simulink library "Equations_of_Motion"  (R2024a)
settings: Solver=VariableStepAuto  StartTime=0.0  StopTime=10.0  RelTol=1e-3
undefined symbols (not defined in the file): g
settings Model: Creator=mahariansyah  LastModifiedBy=mahariansyah

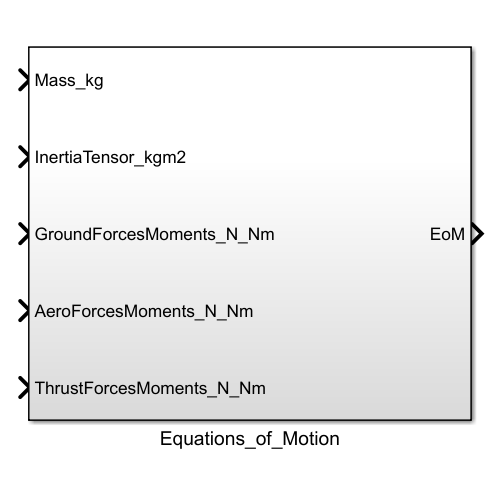
[thumbnail: Simulink's stored preview of the top-level diagram]
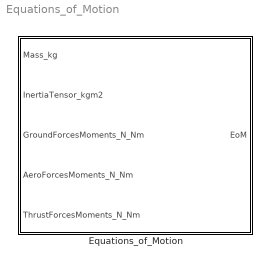
== system Equations_of_Motion ==
  Equations_of_Motion : Subsystem

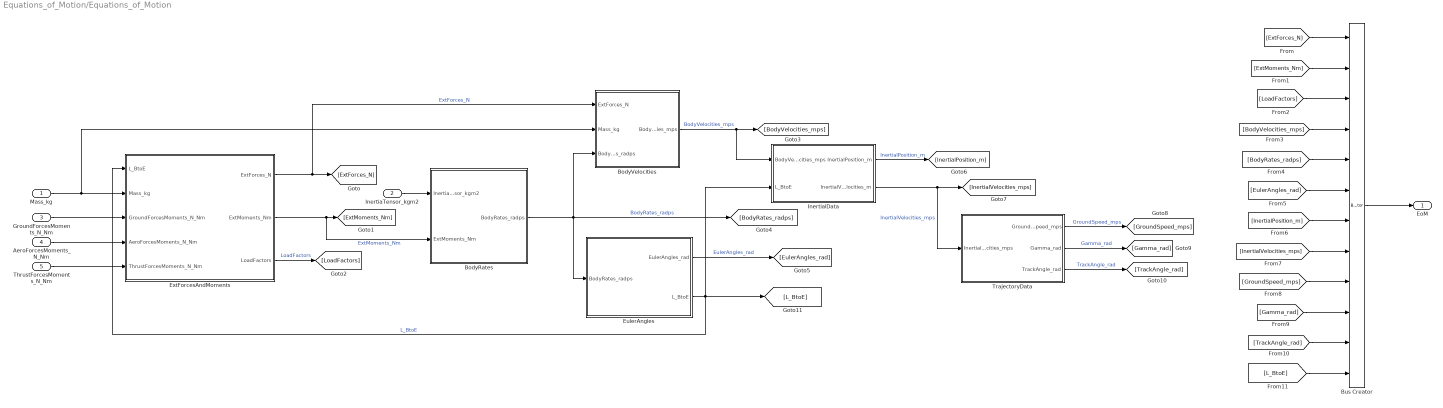
== system Equations_of_Motion/Equations_of_Motion ==
  Mass_kg : Inport
  InertiaTensor_kgm2 : Inport  Port=2
  GroundForcesMoments_N_Nm : Inport  Port=3
  AeroForcesMoments_N_Nm : Inport  Port=4
  ThrustForcesMoments_N_Nm : Inport  Port=5
  BodyRates : Subsystem
  BodyVelocities : Subsystem
  Bus Creator : BusCreator  Inputs=12
  EulerAngles : Subsystem
  ExtForcesAndMoments : Subsystem
  InertialData : Subsystem
  TrajectoryData : Subsystem
  EoM : Outport
  wires:
  [L_BtoE] -> Bus Creator/12
  ExtForcesAndMoments/1(ExtForces_N) -> [ExtForces_N], BodyVelocities/1(ExtForces_N)  "ExtForces_N"
  InertiaTensor_kgm2/1 -> BodyRates/1(InertiaTensor_kgm2)
  Mass_kg/1 -> BodyVelocities/2(Mass_kg), ExtForcesAndMoments/2(Mass_kg)
  Bus Creator/1 -> EoM/1
  BodyVelocities/1(BodyVelocities_mps) -> [BodyVelocities_mps], InertialData/1(BodyVelocities_mps)  "BodyVelocities_mps"
  EulerAngles/2(L_BtoE) -> InertialData/2(L_BtoE), ExtForcesAndMoments/1(L_BtoE), [L_BtoE]  "L_BtoE"
  BodyRates/1(BodyRates_radps) -> BodyVelocities/3(BodyRates_radps), EulerAngles/1(BodyRates_radps), [BodyRates_radps]  "BodyRates_radps"
  [GroundSpeed_mps] -> Bus Creator/9
  AeroForcesMoments_N_Nm/1 -> ExtForcesAndMoments/4(AeroForcesMoments_N_Nm)
  ExtForcesAndMoments/2(ExtMoments_Nm) -> [ExtMoments_Nm], BodyRates/2(ExtMoments_Nm)  "ExtMoments_Nm"
  [TrackAngle_rad] -> Bus Creator/11
  GroundForcesMoments_N_Nm/1 -> ExtForcesAndMoments/3(GroundForcesMoments_N_Nm)
  [BodyRates_radps] -> Bus Creator/5
  [ExtForces_N] -> Bus Creator/1
  [ExtMoments_Nm] -> Bus Creator/2
  [BodyVelocities_mps] -> Bus Creator/4
  [InertialPosition_m] -> Bus Creator/7
  [InertialVelocities_mps] -> Bus Creator/8
  TrajectoryData/2(Gamma_rad) -> [Gamma_rad]  "Gamma_rad"
  ThrustForcesMoments_N_Nm/1 -> ExtForcesAndMoments/5(ThrustForcesMoments_N_Nm)
  InertialData/2(InertialVelocities_m) -> [InertialVelocities_mps], TrajectoryData/1(InertialVelocities_mps)  "InertialVelocities_mps"
  EulerAngles/1(EulerAngles_rad) -> [EulerAngles_rad]  "EulerAngles_rad"
  [LoadFactors] -> Bus Creator/3
  [EulerAngles_rad] -> Bus Creator/6
  [Gamma_rad] -> Bus Creator/10
  TrajectoryData/3(TrackAngle_rad) -> [TrackAngle_rad]  "TrackAngle_rad"
  TrajectoryData/1(GroundSpeed_mps) -> [GroundSpeed_mps]  "GroundSpeed_mps"
  ExtForcesAndMoments/3(LoadFactors) -> [LoadFactors]  "LoadFactors"
  InertialData/1(InertialPosition_m) -> [InertialPosition_m]  "InertialPosition_m"

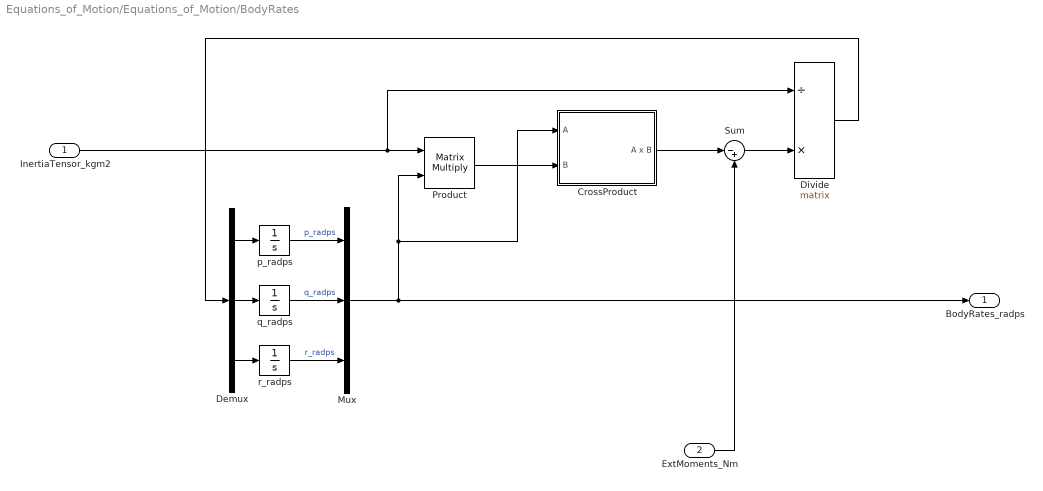
== system Equations_of_Motion/Equations_of_Motion/BodyRates ==
  InertiaTensor_kgm2 : Inport
  ExtMoments_Nm : Inport  Port=2
  CrossProduct : Subsystem
  Demux : Demux  Outputs=3
  Divide : Product  Inputs=/*  Multiplication=Matrix(*)
  Mux : Mux  Inputs=3
  Product : Product  Multiplication=Matrix(*)
  Sum : Sum  Inputs=|-+
  p_radps : Integrator  ContinuousStateAttributes='p_radps'
  q_radps : Integrator  ContinuousStateAttributes='q_radps'
  r_radps : Integrator  ContinuousStateAttributes='r_radps'
  BodyRates_radps : Outport
  wires:
  Demux/1 -> p_radps/1
  Sum/1 -> Divide/2
  q_radps/1 -> Mux/2  "q_radps"
  Demux/2 -> q_radps/1
  Product/1 -> CrossProduct/2(B)
  r_radps/1 -> Mux/3  "r_radps"
  CrossProduct/1(A x B) -> Sum/1
  InertiaTensor_kgm2/1 -> Divide/1, Product/1
  p_radps/1 -> Mux/1  "p_radps"
  Mux/1 -> BodyRates_radps/1, CrossProduct/1(A), Product/2
  Demux/3 -> r_radps/1
  Divide/1 -> Demux/1
  ExtMoments_Nm/1 -> Sum/2

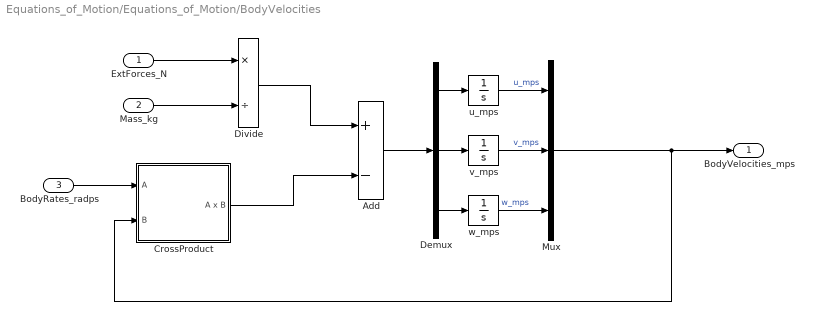
== system Equations_of_Motion/Equations_of_Motion/BodyVelocities ==
  ExtForces_N : Inport
  Mass_kg : Inport  Port=2
  BodyRates_radps : Inport  Port=3
  Add : Sum  Inputs=+-
  CrossProduct : Subsystem
  Demux : Demux  Outputs=3
  Divide : Product  Inputs=*/
  Mux : Mux  Inputs=3
  u_mps : Integrator  ContinuousStateAttributes='u_mps'
  v_mps : Integrator  ContinuousStateAttributes='v_mps'
  w_mps : Integrator  ContinuousStateAttributes='w_mps'
  BodyVelocities_mps : Outport
  wires:
  w_mps/1 -> Mux/3  "w_mps"
  u_mps/1 -> Mux/1  "u_mps"
  v_mps/1 -> Mux/2  "v_mps"
  Demux/2 -> v_mps/1
  Add/1 -> Demux/1
  CrossProduct/1(A x B) -> Add/2
  Divide/1 -> Add/1
  Demux/3 -> w_mps/1
  Mux/1 -> BodyVelocities_mps/1, CrossProduct/2(B)
  Demux/1 -> u_mps/1
  Mass_kg/1 -> Divide/2
  ExtForces_N/1 -> Divide/1
  BodyRates_radps/1 -> CrossProduct/1(A)

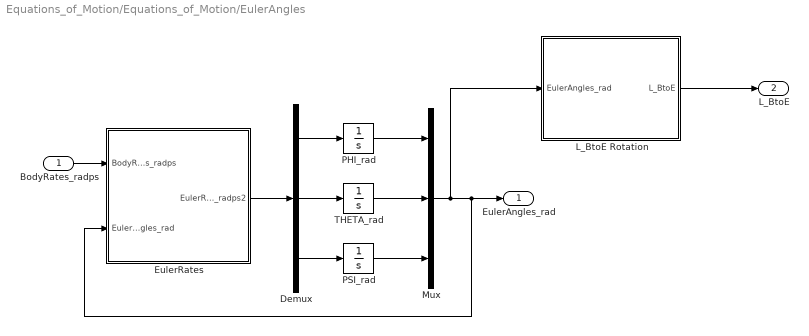
== system Equations_of_Motion/Equations_of_Motion/EulerAngles ==
  BodyRates_radps : Inport
  Demux : Demux  Outputs=3
  EulerRates : Subsystem
  L_BtoE Rotation : Subsystem
  Mux : Mux  Inputs=3
  PHI_rad : Integrator  ContinuousStateAttributes='PHI_rad'
  PSI_rad : Integrator  ContinuousStateAttributes='PSI_rad'
  THETA_rad : Integrator  ContinuousStateAttributes='THETA_rad'
  EulerAngles_rad : Outport
  L_BtoE : Outport  Port=2
  wires:
  EulerRates/1(EulerRates_radps2) -> Demux/1
  Demux/3 -> PSI_rad/1
  Demux/2 -> THETA_rad/1
  THETA_rad/1 -> Mux/2
  L_BtoE Rotation/1(L_BtoE) -> L_BtoE/1
  PSI_rad/1 -> Mux/3
  Demux/1 -> PHI_rad/1
  PHI_rad/1 -> Mux/1
  Mux/1 -> EulerRates/2(EulerAngles_rad), EulerAngles_rad/1, L_BtoE Rotation/1(EulerAngles_rad)
  BodyRates_radps/1 -> EulerRates/1(BodyRates_radps)

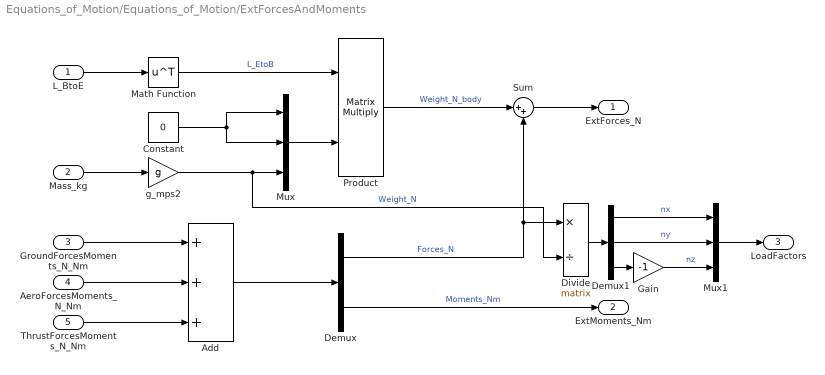
== system Equations_of_Motion/Equations_of_Motion/ExtForcesAndMoments ==
  L_BtoE : Inport
  Mass_kg : Inport  Port=2
  GroundForcesMoments_N_Nm : Inport  Port=3
  AeroForcesMoments_N_Nm : Inport  Port=4
  ThrustForcesMoments_N_Nm : Inport  Port=5
  Add : Sum  Inputs=+++
  Constant : Constant  Value=0
  Demux : Demux  Outputs=2
  Demux1 : Demux  Outputs=3
  Divide : Product  Inputs=*/  Multiplication=Matrix(*)
  Gain : Gain  Gain=-1
  Math Function : Math  Operator=transpose
  Mux : Mux  Inputs=3
  Mux1 : Mux  Inputs=3
  Product : Product  Multiplication=Matrix(*)
  Sum : Sum  Inputs=|++
  g_mps2 : Gain  Gain=g
  ExtForces_N : Outport
  ExtMoments_Nm : Outport  Port=2
  LoadFactors : Outport  Port=3
  wires:
  Demux1/1 -> Mux1/1  "nx"
  Constant/1 -> Mux/2, Mux/1
  Math Function/1 -> Product/1  "L_EtoB"
  Sum/1 -> ExtForces_N/1
  Add/1 -> Demux/1
  g_mps2/1 -> Mux/3, Divide/2  "Weight_N"
  Demux/1 -> Sum/2, Divide/1  "Forces_N"
  Mass_kg/1 -> g_mps2/1
  Divide/1 -> Demux1/1
  Demux1/3 -> Gain/1
  L_BtoE/1 -> Math Function/1
  Mux1/1 -> LoadFactors/1
  Mux/1 -> Product/2
  Demux1/2 -> Mux1/2  "ny"
  Gain/1 -> Mux1/3  "nz"
  ThrustForcesMoments_N_Nm/1 -> Add/3
  GroundForcesMoments_N_Nm/1 -> Add/1
  AeroForcesMoments_N_Nm/1 -> Add/2
  Demux/2 -> ExtMoments_Nm/1  "Moments_Nm"
  Product/1 -> Sum/1  "Weight_N_body"

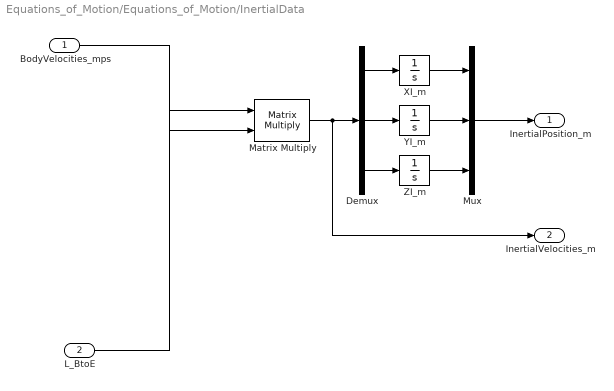
== system Equations_of_Motion/Equations_of_Motion/InertialData ==
  BodyVelocities_mps : Inport
  L_BtoE : Inport  Port=2
  Demux : Demux  Outputs=3
  Matrix Multiply : Product  Multiplication=Matrix(*)
  Mux : Mux  Inputs=3
  XI_m : Integrator  ContinuousStateAttributes="\"XI_m\""
  YI_m : Integrator  ContinuousStateAttributes="\"YI_m\""
  ZI_m : Integrator  ContinuousStateAttributes="\"ZI_m\""
  InertialPosition_m : Outport
  InertialVelocities_m : Outport  Port=2
  wires:
  L_BtoE/1 -> Matrix Multiply/1
  Matrix Multiply/1 -> InertialVelocities_m/1, Demux/1
  YI_m/1 -> Mux/2
  Demux/1 -> XI_m/1
  ZI_m/1 -> Mux/3
  Mux/1 -> InertialPosition_m/1
  XI_m/1 -> Mux/1
  Demux/3 -> ZI_m/1
  Demux/2 -> YI_m/1
  BodyVelocities_mps/1 -> Matrix Multiply/2

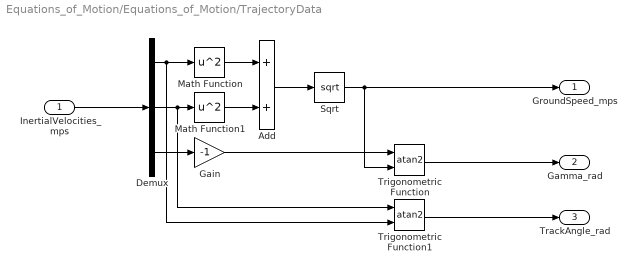
== system Equations_of_Motion/Equations_of_Motion/TrajectoryData ==
  InertialVelocities_mps : Inport
  Add : Sum
  Demux : Demux  Outputs=3
  Gain : Gain  Gain=-1
  Math Function : Math  Operator=square
  Math Function1 : Math  Operator=square
  Sqrt : Sqrt
  Trigonometric Function : Trigonometry  Operator=atan2
  Trigonometric Function1 : Trigonometry  Operator=atan2
  GroundSpeed_mps : Outport
  Gamma_rad : Outport  Port=2
  TrackAngle_rad : Outport  Port=3
  wires:
  Add/1 -> Sqrt/1
  Math Function1/1 -> Add/2
  Math Function/1 -> Add/1
  Demux/1 -> Trigonometric Function1/2, Math Function/1
  Trigonometric Function1/1 -> TrackAngle_rad/1
  Gain/1 -> Trigonometric Function/1
  Demux/2 -> Trigonometric Function1/1, Math Function1/1
  InertialVelocities_mps/1 -> Demux/1
  Sqrt/1 -> GroundSpeed_mps/1, Trigonometric Function/2
  Demux/3 -> Gain/1
  Trigonometric Function/1 -> Gamma_rad/1

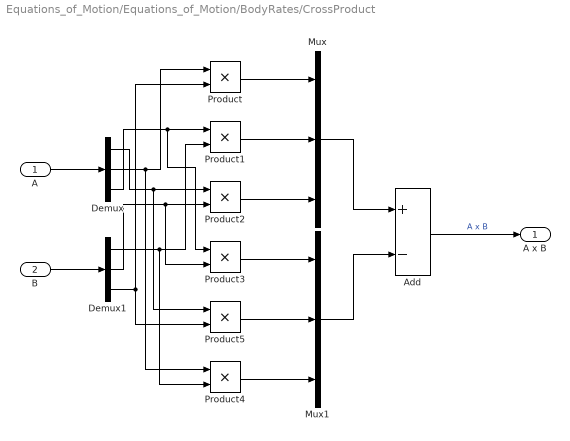
== system Equations_of_Motion/Equations_of_Motion/BodyRates/CrossProduct ==
  A : Inport
  B : Inport  Port=2
  Add : Sum  Inputs=+-
  Demux : Demux  Outputs=3
  Demux1 : Demux  Outputs=3
  Mux : Mux  Inputs=3
  Mux1 : Mux  Inputs=3
  Product{,1..5} (6 alike) : Product
  A x B : Outport
  wires:
  Demux1/3 -> Product5/2, Product/2
  Demux/1 -> Product5/1, Product2/1
  Demux/3 -> Product3/1, Product1/1
  Product2/1 -> Mux/3
  Product5/1 -> Mux1/2
  Demux1/2 -> Product3/2, Product2/2
  Mux1/1 -> Add/2
  Demux1/1 -> Product4/2, Product1/2
  Demux/2 -> Product4/1, Product/1
  Product4/1 -> Mux1/3
  Product/1 -> Mux/1
  Product1/1 -> Mux/2
  Mux/1 -> Add/1
  A/1 -> Demux/1
  Product3/1 -> Mux1/1
  B/1 -> Demux1/1
  Add/1 -> A x B/1  "A x B"

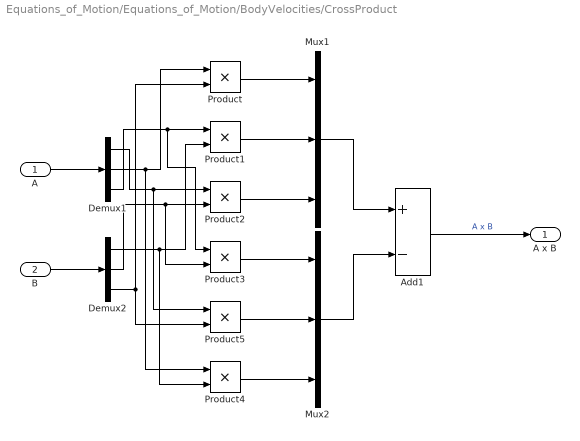
== system Equations_of_Motion/Equations_of_Motion/BodyVelocities/CrossProduct ==
  A : Inport
  B : Inport  Port=2
  Add1 : Sum  Inputs=+-
  Demux1 : Demux  Outputs=3
  Demux2 : Demux  Outputs=3
  Mux1 : Mux  Inputs=3
  Mux2 : Mux  Inputs=3
  Product{,1..5} (6 alike) : Product
  A x B : Outport
  wires:
  Add1/1 -> A x B/1  "A x B"
  A/1 -> Demux1/1
  B/1 -> Demux2/1
  Product1/1 -> Mux1/2
  Demux1/2 -> Product4/1, Product/1
  Product4/1 -> Mux2/3
  Demux2/1 -> Product4/2, Product1/2
  Product/1 -> Mux1/1
  Product5/1 -> Mux2/2
  Product3/1 -> Mux2/1
  Mux1/1 -> Add1/1
  Mux2/1 -> Add1/2
  Product2/1 -> Mux1/3
  Demux2/2 -> Product3/2, Product2/2
  Demux1/1 -> Product5/1, Product2/1
  Demux1/3 -> Product3/1, Product1/1
  Demux2/3 -> Product5/2, Product/2

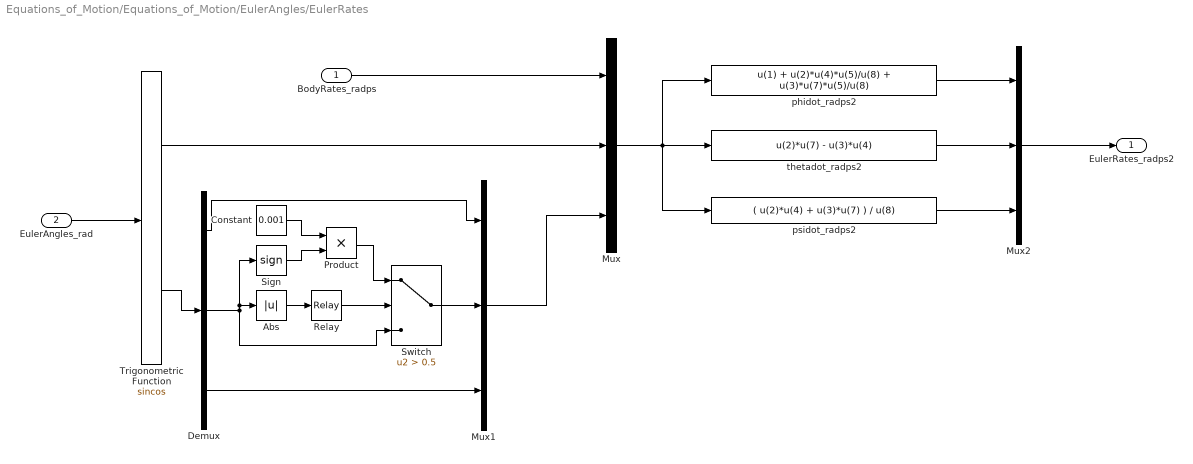
== system Equations_of_Motion/Equations_of_Motion/EulerAngles/EulerRates ==
  BodyRates_radps : Inport
  EulerAngles_rad : Inport  Port=2
  Abs : Abs  SaturateOnIntegerOverflow=off
  Constant : Constant  Value=0.001
  Demux : Demux  Outputs=3
  Mux : Mux  Inputs=3
  Mux1 : Mux  Inputs=3
  Mux2 : Mux  Inputs=3
  Product : Product
  Relay : Relay  OnSwitchValue=0.001  OffSwitchValue=0  OnOutputValue=0  OffOutputValue=1
  Sign : Signum
  Switch : Switch  Criteria=u2 > Threshold  Threshold=0.5  SaturateOnIntegerOverflow=off  InputSameDT=off
  Trigonometric Function : Trigonometry  Operator=sincos
  phidot_radps2 : Fcn  Expr=u(1) + u(2)*u(4)*u(5)/u(8) + u(3)*u(7)*u(5)/u(8)
  psidot_radps2 : Fcn  Expr=( u(2)*u(4) + u(3)*u(7) ) / u(8)
  thetadot_radps2 : Fcn  Expr=u(2)*u(7) - u(3)*u(4)
  EulerRates_radps2 : Outport
  wires:
  Mux1/1 -> Mux/3
  EulerAngles_rad/1 -> Trigonometric Function/1
  Abs/1 -> Relay/1
  Demux/2 -> Sign/1, Abs/1, Switch/3
  phidot_radps2/1 -> Mux2/1
  Demux/1 -> Mux1/1
  Switch/1 -> Mux1/2
  Mux/1 -> phidot_radps2/1, psidot_radps2/1, thetadot_radps2/1
  BodyRates_radps/1 -> Mux/1
  psidot_radps2/1 -> Mux2/3
  Trigonometric Function/2 -> Demux/1
  Trigonometric Function/1 -> Mux/2
  Demux/3 -> Mux1/3
  thetadot_radps2/1 -> Mux2/2
  Relay/1 -> Switch/2
  Sign/1 -> Product/2
  Constant/1 -> Product/1
  Product/1 -> Switch/1
  Mux2/1 -> EulerRates_radps2/1

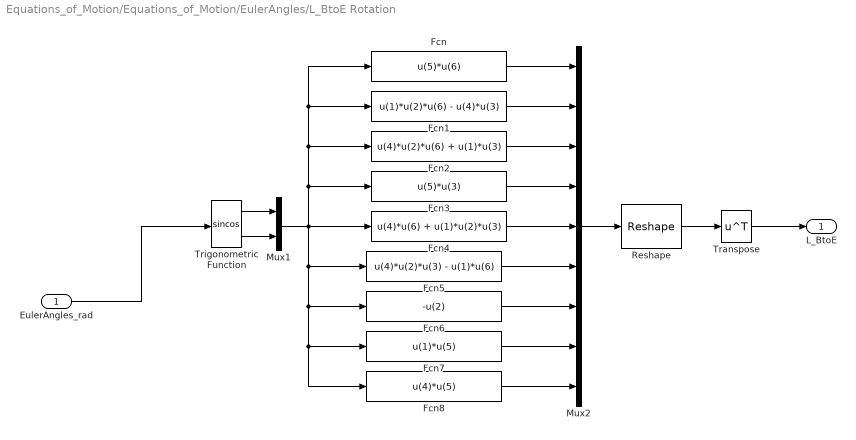
== system Equations_of_Motion/Equations_of_Motion/EulerAngles/L_BtoE Rotation ==
  EulerAngles_rad : Inport
  Fcn : Fcn  Expr=u(5)*u(6)
  Fcn1 : Fcn  Expr=u(1)*u(2)*u(6) - u(4)*u(3)
  Fcn2 : Fcn  Expr=u(4)*u(2)*u(6) + u(1)*u(3)
  Fcn3 : Fcn  Expr=u(5)*u(3)
  Fcn4 : Fcn  Expr=u(4)*u(6) + u(1)*u(2)*u(3)
  Fcn5 : Fcn  Expr=u(4)*u(2)*u(3) - u(1)*u(6)
  Fcn6 : Fcn  Expr=-u(2)
  Fcn7 : Fcn  Expr=u(1)*u(5)
  Fcn8 : Fcn  Expr=u(4)*u(5)
  Mux1 : Mux  Inputs=2
  Mux2 : Mux  Inputs=9
  Reshape : Reshape  OutputDimensionality=Customize  OutputDimensions=[3,3]
  Transpose : Math  Operator=transpose
  Trigonometric Function : Trigonometry  Operator=sincos
  L_BtoE : Outport
  wires:
  Fcn3/1 -> Mux2/4
  Trigonometric Function/1 -> Mux1/1
  EulerAngles_rad/1 -> Trigonometric Function/1
  Trigonometric Function/2 -> Mux1/2
  Fcn4/1 -> Mux2/5
  Fcn6/1 -> Mux2/7
  Mux1/1 -> Fcn4/1, Fcn3/1, Fcn2/1, Fcn1/1, Fcn/1, Fcn5/1, Fcn8/1, Fcn7/1, Fcn6/1
  Fcn1/1 -> Mux2/2
  Reshape/1 -> Transpose/1
  Fcn/1 -> Mux2/1
  Transpose/1 -> L_BtoE/1
  Fcn5/1 -> Mux2/6
  Fcn8/1 -> Mux2/9
  Fcn2/1 -> Mux2/3
  Fcn7/1 -> Mux2/8
  Mux2/1 -> Reshape/1
